simulink model "Nonlinear_ILC"  (R2017a)
settings: Solver=FixedStepAuto  StartTime=0.0  StopTime=10.0  FixedStep=T  RelTol=1e-3
undefined symbols (not defined in the file or in its folder): Gam
settings Model: Creator=capn  LastModifiedBy=capn
settings DebuggingCC: AlgebraicLoopMsg=none

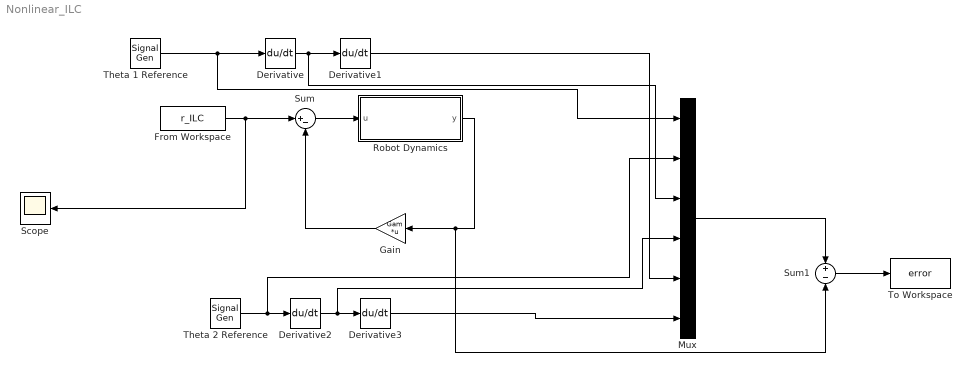
== system Nonlinear_ILC ==
  Derivative{,1..3} (4 alike) : Derivative
  From Workspace : FromWorkspace  VariableName=r_ILC  SampleTime=0
  Gain : Gain  Gain=Gam  Multiplication=Matrix(K*u)
  Mux : Mux  Inputs=6
  Robot Dynamics : Subsystem
  Scope : Scope
  Sum : Sum  Inputs=|+-
  Sum1 : Sum  Inputs=+-
  Theta 1 Reference : SignalGenerator  Frequency=2  Units=rad/sec
  Theta 2 Reference : SignalGenerator  Units=rad/sec
  To Workspace : ToWorkspace  VariableName=error  SampleTime=-1
  wires:
  Robot Dynamics/1(y) -> Sum1/2, Gain/1
  Gain/1 -> Sum/2
  Sum/1 -> Robot Dynamics/1("u ")
  From Workspace/1 -> Scope/1, Sum/1
  Theta 1 Reference/1 -> Mux/1, Derivative/1
  Derivative/1 -> Mux/3, Derivative1/1
  Theta 2 Reference/1 -> Mux/2, Derivative2/1
  Derivative2/1 -> Mux/4, Derivative3/1
  Derivative1/1 -> Mux/5
  Derivative3/1 -> Mux/6
  Mux/1 -> Sum1/1
  Sum1/1 -> To Workspace/1

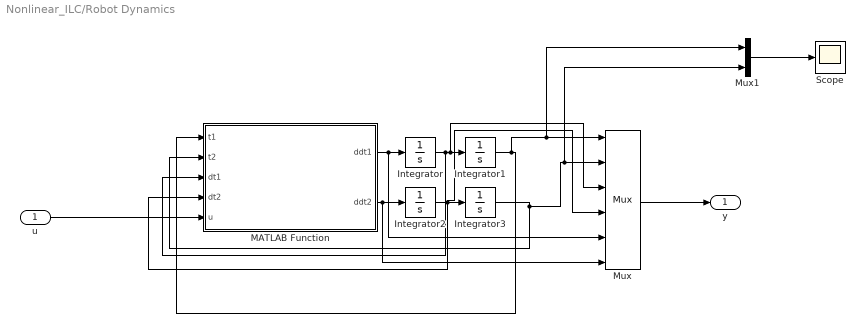
== system Nonlinear_ILC/Robot Dynamics ==
  "u " : Inport  PortDimensions=2
  Integrator{,1..3} (4 alike) : Integrator
  MATLAB Function : MATLAB Function
  Mux : Mux  Inputs=6
  Mux1 : Mux  Inputs=2
  Scope : Scope
  y : Outport
  wires:
  Integrator3/1 -> Mux1/2, Mux/2, MATLAB Function/2(t2)
  Integrator2/1 -> Mux/4, MATLAB Function/4(dt2), Integrator3/1
  Integrator1/1 -> Mux1/1, Mux/1, MATLAB Function/1(t1)
  MATLAB Function/2(ddt2) -> Mux/6, Integrator2/1
  MATLAB Function/1(ddt1) -> Mux/5, Integrator/1
  Integrator/1 -> MATLAB Function/3(dt1), Mux/3, Integrator1/1
  "u "/1 -> MATLAB Function/5(u)
  Mux/1 -> y/1
  Mux1/1 -> Scope/1

== matlab function Nonlinear_ILC/Robot Dynamics/MATLAB Function ==
  data: t1 input size=1; t2 input size=1; dt1 input size=1; dt2 input size=1; u input size=2; ddt1 output size=1; ddt2 output size=1
function [ddt1,ddt2] = fcn(t1,t2,dt1,dt2,u)
A = [0.54+0.27*cos(t2) 0.135+0.135*cos(t2);0.135+0.135*cos(t2) 0.135];
B = [0.135*sin(t2) 0;-0.27*sin(t2) -.135*sin(t2)*dt2];
C = [13.1625*sin(t1)+4.3875*sin(t1+t2);4.3875*sin(t1+t2)];

ddx = inv(A)*(u-B*[dt1;dt2]-C);
ddt1 = ddx(1);
ddt2 = ddx(2);
